simulink model "RobotX_FullSystemSep20"  (R2014a)
settings: Solver=FixedStepDiscrete  StartTime=0.0  StopTime=inf  FixedStep=.25  RelTol=1e-3
undefined symbols (not defined in the file): Com1, Com2, Com3, Com4, DiscIntNeverNeededParam, standard
libraries: simulink x11, xpcseriallib x11, slrtlib x3, speedgoatlib x1, speedgoatlib_IO102 x1
(part 4 of 4)

== matlab function RobotX_FullSystemSep20/Main FSM/Termination/GPSMove ==
  data: GoalNED input; X input; valid output; Y input; Psi input; pts output
function [valid,pts] = GPSmove(GoalNED,X,Y,Psi)
%Written by Dylan DeGaetano on September 1, 2014
%Last edited by: Anderson Lebbad
%
%This function will go to a given NED cooridnate, last edit changed the
%goal pt and variable names

persistent Sample
if isempty(Sample)
Sample = 0;
end

pts = zeros(8,2);
%$Distance to object in meters

if Sample == 0
    pts(1,1) = X+5*cos(Psi*pi/180);
    pts(1,2) = Y+5*cos(Psi*pi/180);
    pts(8,1) = GoalNED(1,1);
    pts(8,2) = GoalNED(1,2);
    pts(2,:) = pts(1,:) +(1*(GoalNED-pts(1,:))/7);
    pts(3,:) = pts(1,:) +(2*(GoalNED-pts(1,:))/7);
    pts(4,:) = pts(1,:) +(3*(GoalNED-pts(1,:))/7);
    pts(5,:) = pts(1,:) +(4*(GoalNED-pts(1,:))/7);
    pts(6,:) = pts(1,:) +(5*(GoalNED-pts(1,:))/7);
    pts(7,:) = pts(1,:) +(6*(GoalNED-pts(1,:))/7);
    Sample = 1; 
    valid = 1;
    
else
    valid = 0;
end

== matlab function RobotX_FullSystemSep20/Main FSM/OD//OA Path/A Star (Held Length) ==
  data: relPose input; Path output; obGrid input; targetPt input
function Path  = AStarHeldLengthDebug( relPose, obGrid, targetPt )
%Written By Anderson Lebbad on August 27, 2014
%Last Edited on:

%This funtion executes an A* method for path planning given the current
%position of the vessel, the target position for the vessel to reach, and
%a map of obstacles to avoid. The A* method is well documented here:
% www.policyalmanac.org/games/aStarTutorial.htm

%% Define list sizes
[m,n] = size(obGrid);
gridPts = m*n;

%Initialize a path output variable
Path = nan(gridPts,2);
%Initialize variable to track if a solution has been found
solution_found = 0;

%Track the XY coordinates of each point to be evaluated
open_list_XY = nan(gridPts,2);
%Track the calculated F, G, and H weights (where G is the movement cost to
%get to the point, H is the Hypothetical cost to reach the target from that
%point before the full path is evaluated, and F is the sum of both G and H
%costs) for the points being evaluated
open_list_FGH = nan(gridPts,3);
%Track the coordinates of the parent for each of the points being evaluated
open_list_parent = nan(gridPts,2);

%Track the XY coordinates of each point that has been fully evaluated
closed_list_XY = nan(gridPts,2);
%Track the parent coordinate of each point that has been fully evaluated
closed_list_parent = nan(gridPts,2);
emptyClosed = find(isnan(closed_list_XY(:,1)));

%Relative indices to neighboring points of the square, to be used for
%evaluating potential candidates for the open list
neighbors_XY = [-1,-1;-1,0;-1,1;0,1;1,1;1,0;1,-1;0,-1];
neighbors_G = [14;10;14;10;14;10;14;10];

%Make the current pose (in the relative coordinates of the field) the first
%point in the open list
open_list_XY(1,:) = relPose;
current_XY = relPose;
%Set movement cost of this point to zero
open_list_FGH(1,2) = 0;
%Calculate hypothetical cost
open_list_FGH(1,3) = 10*(abs(targetPt(1)-relPose(1))+abs(targetPt(2)-relPose(2)));
%Sum is full cost
open_list_FGH(1,1) = open_list_FGH(1,2) + open_list_FGH(1,3);

%Create a list of invalid pts
%obstacles are invalid
[row, col] = find(obGrid == -1);
%outside the edges are invalid
left = [0:m+1;zeros(1,m+2)]';
right = [0:m+1;(n+1)*ones(1,m+2)]';
bottom = [zeros(1,n);1:n]';
top = [(m+1)*ones(1,n);1:n]';
invalid_pts = [row,col;left;right;bottom;top];
invalid_pts = sortrows(invalid_pts);
%Loop while there are points on the open list
while sum(~isnan(open_list_XY(:,1))) >= 1
    %% Current Square
    
    %Find the lowest F cost square on the open list, checking newer entries
    %over older. This is done by flipping the list up/down to get newer
    %entries to evaluate first. This is marked as the current square
    [~,idxI] = min(flipud(open_list_FGH(:,1)));
    CurrentSquare = gridPts - idxI(1) + 1;
    current_XY = open_list_XY(CurrentSquare,:);
    current_G = open_list_FGH(CurrentSquare,2);
    
    %Find the first empty element in the closed list, and replace the place
    %holder with the information for the current square
    emptyClosed = find(isnan(closed_list_XY(:,1)));
    closed_list_XY(emptyClosed(1),:) = current_XY;
    closed_list_parent(emptyClosed(1),:) = open_list_parent(CurrentSquare,:);
    %Remove the current square from the open list now that it is on the
    %closed list
    open_list_XY(CurrentSquare,:) = NaN;
    open_list_FGH(CurrentSquare,:) = NaN;
    open_list_parent(CurrentSquare,:) = NaN;
    
    %If the current point that just got added to the closed list is the
    %target point, exit the loop because a complete path can be traced
    if (current_XY(1) == targetPt(1)) && (current_XY(2) == targetPt(2))
        solution_found = 1;
        break
    end
    
    %% Check adjacent squares
    
    %Create a list of points around the current point and check their G
    %value
    rel_list_XY = [neighbors_XY(:,1)+current_XY(1) neighbors_XY(:,2)+current_XY(2)];
    rel_list_G = neighbors_G + current_G;
    rel_list_H = 10*(abs(targetPt(1)-rel_list_XY(:,1))+abs(targetPt(2)-rel_list_XY(:,2)));
    rel_list_F = rel_list_G + rel_list_H;
    
    %% Check walkable / on closed list
    
    %Order closed list for finding relative list points on it
    closed_list_XY_sorted = sortrows(closed_list_XY);
    %Mark members of relative list if on closed list
    on_closed = ismember(rel_list_XY,closed_list_XY_sorted,'rows');
    rel_list_XY(on_closed,:) = NaN;
    rel_list_F(on_closed) = NaN;
    rel_list_G(on_closed) = NaN;
    rel_list_H(on_closed) = NaN;
    %Check to see if members of relative list are either obstacles or out
    %of bounds
    invalid = ismember(rel_list_XY,invalid_pts,'rows');
    rel_list_XY(invalid,:) = NaN;
    rel_list_F(invalid) = NaN;
    rel_list_G(invalid) = NaN;
    rel_list_H(invalid) = NaN;
    valid = ~isnan(rel_list_XY(:,1));
    validIdx = find(valid);
    
    %% Calculate F and H, and add penalty weights to G scores
    
    if ~isempty(rel_list_XY)
        rel_list_G(valid) = rel_list_G(valid) + 20.*obGrid(rel_list_XY(valid,1)+m*(rel_list_XY(valid,2)-1));
        rel_list_F(valid) = rel_list_G(valid) + rel_list_H(valid);
        
        %% Check if on open list, if not add to it
        
        %Order open list for finding relative list points on it
        [open_list_XY_sorted, idx] = sortrows(open_list_XY);
        %Check to see if relative list points are on open list
        [rel_on_open, open_on_rel_list] = ismember(rel_list_XY(valid,:),open_list_XY_sorted,'rows');
        rel_not_on_open = validIdx(~rel_on_open);
        rel_on_open = validIdx(rel_on_open);
        %Only care about indices that are actually found, remove the ones that
        %aren't
        open_on_rel = idx(open_on_rel_list(open_on_rel_list ~= 0));
        %Whichever points that are not on the open list are
        %added to the open list (in the first available empty slots)
        num_not_on_open = length(rel_not_on_open);
        num_on_open = length(rel_on_open);
        emptyOpen = find(isnan(open_list_XY(:,1)));
        if num_not_on_open >= 1
            open_list_XY(emptyOpen(1:num_not_on_open),:) = rel_list_XY(rel_not_on_open,:);
            open_list_FGH(emptyOpen(1:num_not_on_open),:) = ...
                [rel_list_F(rel_not_on_open) rel_list_G(rel_not_on_open) rel_list_H(rel_not_on_open)];
            open_list_parent(emptyOpen(1:num_not_on_open),1) = current_XY(1);
            open_list_parent(emptyOpen(1:num_not_on_open),2) = current_XY(2);
            %Remove members of the relative list that were just put on the open
            %list (only care about the F and G, the XY and H are not updated past
            %this point)
            rel_list_F(~rel_on_open) = NaN;
            rel_list_G(~rel_on_open) = NaN;
        end
        
        %% Check G cost of rest to see if it should be updated
        
        if num_on_open >= 1
            %Find the G values of the points that are on the open list and compare
            %them to the G values for the same points on the relative list. Track
            %which G values are lower on the relative list
            lower_G_list = rel_list_G(rel_on_open) < open_list_FGH(open_on_rel,2);
            rel_idx = find(rel_on_open);
            lower_G = rel_idx(lower_G_list);
            %Replace the G and F values with the new lower ones, and update parent
            open_list_FGH(open_on_rel(lower_G_list),1:2) = [rel_list_F(lower_G) rel_list_G(lower_G)];
            open_list_parent(open_on_rel(lower_G_list),1) = current_XY(1);
            open_list_parent(open_on_rel(lower_G_list),2) = current_XY(2);
        end
        
    end
    
    %% Organize list for searching
    
    %Negates the F and H cost for to be able to descending rowsort, then negates
    %back to original values
    open_list_FGH = -open_list_FGH;
    [open_list_FGH,idx] = sortrows(open_list_FGH,[1 3]); %Sort focusing on F first, then H
    open_list_FGH = -open_list_FGH;
    open_list_XY = open_list_XY(idx,:);
    open_list_parent = open_list_parent(idx,:);
    
end

%% If solution is found, generate path

%Generate path by recursively checking parent values
if solution_found
    %Create a list of the path points, for organizational purposes for
    %outputting later
    PathList = Path;
    %Set first element as current position (the goal point)
    PathList(1,:) = current_XY;
    %Track current square's location on closed list
    CurrentSquareClosed = emptyClosed(1);
    %Create an incrementing variable for path elements
    next_index = 2;
    %Loop until there is no parent square (start square)
    while ~isnan(closed_list_parent(CurrentSquareClosed))
        %Next path element is the current element's parent
        PathList(next_index,:) = closed_list_parent(CurrentSquareClosed,:);
        %Order closed list for finding parents on it
        [closed_list_XY_sorted, idx] = sortrows(closed_list_XY);
        %Find the next element and make it the current element
        [~,locs] = ismember(closed_list_parent(CurrentSquareClosed,:),closed_list_XY_sorted,'rows');
        CurrentSquareClosed = idx(locs(1));
        %Increment the next index
        next_index = next_index + 1;
    end
    %Get the length of the path
    PathLength = next_index-1;
    %Path list is from finish to start, so flip and output
    Path(1:PathLength,:) = PathList(PathLength:-1:1,:);
end

end
